simulink model "motorsPID_MD"  (R2018a)
settings: Solver=ode45  StartTime=0.0  StopTime=Tsim  RelTol=1e-3  EnableMultiTasking=on
values from neighbouring files (symbols this model uses):
  thetai = 0    [AjusteC.m]    (also in AjusteC2.m; AjusteCVaryReal.m; simula_robo.m = 1.57079632679)
  Ts = 0.1    [AjusteC.m]    (also in AjusteC2.m; AjusteCVaryReal.m; GenPath.m; GenPath2.m)
  vmax = 0.8    [AjusteC.m]    (also in AjusteC2.m; AjusteCVaryReal.m; simula_robo.m)
  vmin = -vmax    (= -0.8)    [AjusteC.m]    (also in AjusteC2.m; AjusteCVaryReal.m; simula_robo.m)
  wmax = 0.8    [AjusteC.m]    (also in AjusteC2.m; AjusteCVaryReal.m; simula_robo.m)
  wmin = -wmax    (= -0.8)    [AjusteC.m]    (also in AjusteC2.m; AjusteCVaryReal.m; simula_robo.m)
  xi = 0    [AjusteC.m]    (also in AjusteC2.m; AjusteCVaryReal.m = 1; simula_robo.m)
  yi = 0    [AjusteC.m]    (also in AjusteC2.m; AjusteCVaryReal.m = -3; simula_robo.m = -0.5)
undefined symbols (not defined in the file or in its folder): DiscIntNeverNeededParam
settings Model: Creator=Thiago  LastModifiedBy=projeto
settings DataIOCC: LimitDataPoints=on  SaveFormat=Array
settings OptimizationCC: LifeSpan=inf
settings DebuggingCC: SFUnexpectedBacktrackingDiag=warning  SFNoUnconditionalDefaultTransitionDiag=warning  SFExecutionAtInitializationDiag=none
settings HardwareCC: ProdBitPerPointer=32  ProdBitPerSizeT=32  ProdBitPerPtrDiffT=32  ProdLargestAtomicFloat=None  ProdIntDivRoundTo=Undefined  ProdEndianess=Unspecified  ProdWordSize=32  ProdHWDeviceType=32-bit Generic
settings ModelReferenceCC: PropagateSignalLabelsOutOfModel=off
settings CodeAppCC: StateflowObjectComments=on
settings GRTTargetCC: TargetLangStandard=C89/C90 (ANSI)  GeneratePreprocessorConditionals=Disable all
settings ConfigComp: CovMetricSettings=dw  CovHtmlReporting=on  CovSaveCumulativeToWorkspaceVar=on  CovSaveSingleToWorkspaceVar=on  CovExternalEMLEnable=off
settings SimscapeCC: SimscapeNormalizeSystem=off
settings ConfigurationSet: Description=SimMechanics 2G

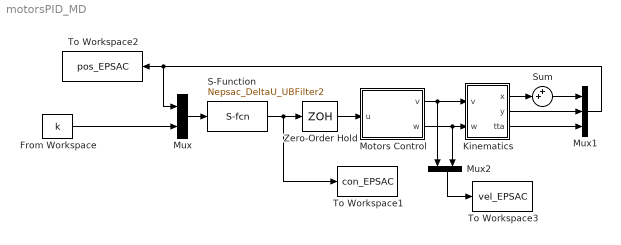
== system motorsPID_MD ==
  From Workspace : FromWorkspace  VariableName=k  SampleTime=Ts
  Kinematics : Subsystem
  Motors Control : Subsystem
  Mux : Mux  Inputs=2
  Mux1 : Mux  Inputs=3
  Mux2 : Mux  Inputs=2
  S-Function : S-Function  FunctionName=Nepsac_DeltaU_UBFilter2  SFunctionDeploymentMode=off  EnableBusSupport=off
  Sum : Sum  Inputs=++|
  To Workspace1 : ToWorkspace  VariableName=con_EPSAC  SaveFormat=Structure With Time  SampleTime=Ts
  To Workspace2 : ToWorkspace  VariableName=pos_EPSAC  SaveFormat=Structure With Time  SampleTime=Ts
  To Workspace3 : ToWorkspace  VariableName=vel_EPSAC  SaveFormat=Structure With Time  SampleTime=Ts
  Zero-Order Hold : ZeroOrderHold  SampleTime=Ts
  wires:
  S-Function/1 -> Zero-Order Hold/1, To Workspace1/1
  Motors Control/1(v) -> Kinematics/1(v), Mux2/1
  Motors Control/2(w) -> Kinematics/2(w), Mux2/2
  Kinematics/2(y) -> Mux1/2
  Kinematics/3(tta) -> Mux1/3
  Mux/1 -> S-Function/1
  Mux1/1 -> Mux/1, To Workspace2/1
  Mux2/1 -> To Workspace3/1
  Zero-Order Hold/1 -> Motors Control/1(u)
  From Workspace/1 -> Mux/2
  Kinematics/1(x) -> Sum/2
  Sum/1 -> Mux1/1

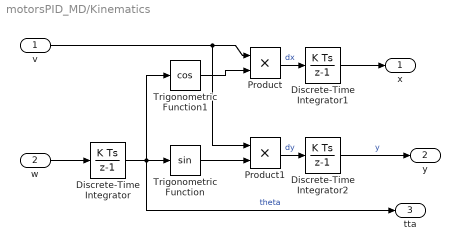
== system motorsPID_MD/Kinematics ==
  v : Inport
  w : Inport  Port=2
  Discrete-Time Integrator : DiscreteIntegrator  InitialCondition=thetai  SampleTime=Ts  ICPrevOutput=DiscIntNeverNeededParam  ICPrevScaledInput=DiscIntNeverNeededParam
  Discrete-Time Integrator1 : DiscreteIntegrator  InitialCondition=xi  SampleTime=Ts  ICPrevOutput=DiscIntNeverNeededParam  ICPrevScaledInput=DiscIntNeverNeededParam
  Discrete-Time Integrator2 : DiscreteIntegrator  InitialCondition=yi  SampleTime=Ts  ICPrevOutput=DiscIntNeverNeededParam  ICPrevScaledInput=DiscIntNeverNeededParam
  Product : Product
  Product1 : Product
  Trigonometric Function : Trigonometry
  Trigonometric Function1 : Trigonometry  Operator=cos
  x : Outport
  y : Outport  Port=2
  tta : Outport  Port=3
  wires:
  v/1 -> Product1/1, Product/1
  Trigonometric Function1/1 -> Product/2
  Product/1 -> Discrete-Time Integrator1/1  "dx"
  Discrete-Time Integrator/1 -> tta/1, Trigonometric Function1/1, Trigonometric Function/1  "theta"
  Discrete-Time Integrator2/1 -> y/1  "y"
  Product1/1 -> Discrete-Time Integrator2/1  "dy"
  Trigonometric Function/1 -> Product1/2
  Discrete-Time Integrator1/1 -> x/1
  w/1 -> Discrete-Time Integrator/1

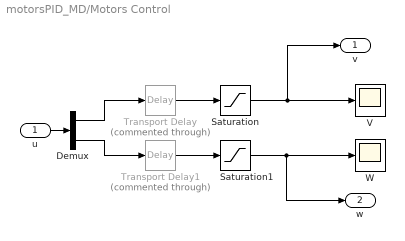
== system motorsPID_MD/Motors Control ==
  u : Inport
  Demux : Demux  Outputs=2
  Saturation : Saturate  UpperLimit=vmax  LowerLimit=vmin
  Saturation1 : Saturate  UpperLimit=wmax  LowerLimit=wmin
  Transport Delay : TransportDelay  Commented=through  DelayTime=0
  Transport Delay1 : TransportDelay  Commented=through  DelayTime=0
  V : Scope
  W : Scope
  v : Outport
  w : Outport  Port=2
  wires:
  Saturation/1 -> v/1, V/1
  Transport Delay1/1 -> Saturation1/1
  Saturation1/1 -> W/1, w/1
  Transport Delay/1 -> Saturation/1
  u/1 -> Demux/1
  Demux/1 -> Transport Delay/1
  Demux/2 -> Transport Delay1/1
